simulink model "flc_case_3"  (R2018a)
settings: Solver=VariableStepAuto  StartTime=0.0  StopTime=30  RelTol=1e-3
libraries: fuzblock x1, simulink x1
settings Model: Creator=Lefteris  LastModifiedBy=Lefteris

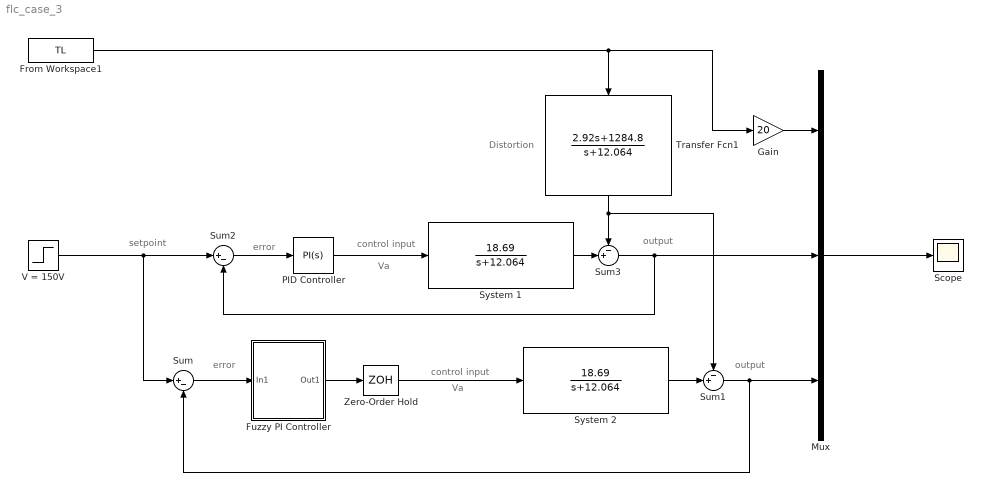
== system flc_case_3 ==
  note: Distortion
  note: setpoint
  note: output
  note: control input
  note: Va
  note: error
  note: error
  note: control input
  note: Va
  note: output
  From Workspace1 : FromWorkspace  VariableName=TL  SampleTime=0.01
  Fuzzy PI Controller : Subsystem
  Gain : Gain  Gain=20
  Mux : Mux  Inputs=3
  PID Controller : simulink/Continuous/PID Controller  Controller=PI  TimeDomain=Continuous-time  SampleTime=-1  IntegratorMethod=Forward Euler  FilterMethod=Forward Euler  Form=Parallel  UseFilter=on  ControllerParametersSource=internal  P=0.31011  I=8.1187  D=0  N=100  InitialConditionSource=internal  InitialConditionForIntegrator=0  InitialConditionForFilter=0  ExternalReset=none  LimitOutput=off  UpperSaturationLimit=inf  LowerSaturationLimit=-inf  LinearizeAsGain=on  AntiWindupMode=none  Kb=1  TrackingMode=off  Kt=1  PParamMin=[]  PParamMax=[]  IParamMin=[]  IParamMax=[]  DParamMin=[]  DParamMax=[]  NParamMin=[]  NParamMax=[]  KbParamMin=[]  KbParamMax=[]  KtParamMin=[]  KtParamMax=[]  POutMin=[]  POutMax=[]  IOutMin=[]  IOutMax=[]  DOutMin=[]  DOutMax=[]  NOutMin=[]  NOutMax=[]  KbOutMin=[]  KbOutMax=[]  KtOutMin=[]  KtOutMax=[]  IntegratorOutMin=[]  IntegratorOutMax=[]  FilterOutMin=[]  FilterOutMax=[]  SumOutMin=[]  SumOutMax=[]  SumI1OutMin=[]  SumI1OutMax=[]  SumI2OutMin=[]  SumI2OutMax=[]  SumI3OutMin=[]  SumI3OutMax=[]  SumDOutMin=[]  SumDOutMax=[]  SaturationOutMin=[]  SaturationOutMax=[]  IntegratorContinuousStateAttributes=''  IntegratorStateMustResolveToSignalObject=off  IntegratorRTWStateStorageClass=Auto  FilterContinuousStateAttributes=''  FilterStateMustResolveToSignalObject=off  FilterRTWStateStorageClass=Auto  DifferentiatorICPrevScaledInput=0  DifferentiatorOutMin=[]  DifferentiatorOutMax=[]  FilterDiffOutCoefMin=[]  FilterDiffOutCoefMax=[]  SumDenOutMin=[]  SumDenOutMax=[]  SumNumOutMin=[]  SumNumOutMax=[]  ReciprocalOutMin=[]  ReciprocalOutMax=[]  DivideOutMin=[]  DivideOutMax=[]  TunerSelectOption=Transfer Function Based (PID Tuner App)
  Scope : Scope
  Sum : Sum  Inputs=|+-
  Sum1 : Sum  Inputs=-+|
  Sum2 : Sum  Inputs=|+-
  Sum3 : Sum  Inputs=-+|
  System 1 : TransferFcn  Numerator=[18.69]  Denominator=[1 12.064]
  System 2 : TransferFcn  Numerator=[18.69]  Denominator=[1 12.064]
  Transfer Fcn1 : TransferFcn  Numerator=[2.92 1284.8]  Denominator=[1 12.064]
  V = 150V : Step  Time=0  After=150  SampleTime=0.01
  Zero-Order Hold : ZeroOrderHold  SampleTime=0.01
  wires:
  Zero-Order Hold/1 -> System 2/1
  Mux/1 -> Scope/1
  Sum/1 -> Fuzzy PI Controller/1(In1)
  V = 150V/1 -> Sum2/1, Sum/1
  Fuzzy PI Controller/1(Out1) -> Zero-Order Hold/1
  System 2/1 -> Sum1/2
  Sum1/1 -> Mux/3, Sum/2
  Sum2/1 -> PID Controller/1
  PID Controller/1 -> System 1/1
  System 1/1 -> Sum3/2
  Sum3/1 -> Sum2/2, Mux/2
  From Workspace1/1 -> Gain/1, Transfer Fcn1/1
  Gain/1 -> Mux/1
  Transfer Fcn1/1 -> Sum1/1, Sum3/1

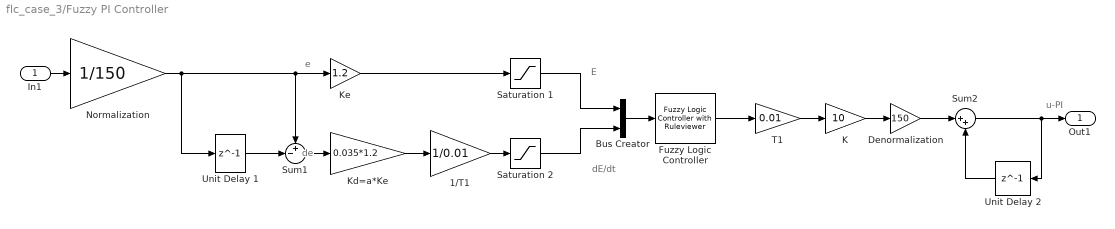
== system flc_case_3/Fuzzy PI Controller ==
  note: u-PI
  note: dE/dt
  note: E
  note: de
  note: e
  In1 : Inport
  1/T1 : Gain  Gain=1/0.01
  Bus Creator : BusCreator  Inputs=2
  "Denormalization " : Gain  Gain=150
  "Fuzzy Logic Controller " : fuzblock/Fuzzy Logic  Controller  with Ruleviewer  fismatrix=fis  Ts=1
  K : Gain  Gain=10
  Kd=a*Ke : Gain  Gain=0.035*1.2
  Ke : Gain  Gain=1.2
  Normalization : Gain  Gain=1/150
  "Saturation 1 " : Saturate  UpperLimit=1  LowerLimit=-1
  "Saturation 2 " : Saturate  UpperLimit=1  LowerLimit=-1
  Sum1 : Sum  Inputs=+-|
  Sum2 : Sum  Inputs=|++
  T1 : Gain  Gain=0.01
  Unit Delay 1 : Delay  DelayLength=1  SampleTime=0.01
  Unit Delay 2 : Delay  DelayLength=1  SampleTime=0.01
  Out1 : Outport
  wires:
  1/T1/1 -> "Saturation 2 "/1
  Kd=a*Ke/1 -> 1/T1/1
  Ke/1 -> "Saturation 1 "/1
  Sum1/1 -> Kd=a*Ke/1
  "Saturation 1 "/1 -> Bus Creator/1
  "Saturation 2 "/1 -> Bus Creator/2
  Unit Delay 2/1 -> Sum2/2
  K/1 -> "Denormalization "/1
  Normalization/1 -> Sum1/1, Ke/1, Unit Delay 1/1
  Unit Delay 1/1 -> Sum1/2
  T1/1 -> K/1
  "Denormalization "/1 -> Sum2/1
  Sum2/1 -> Unit Delay 2/1, Out1/1
  In1/1 -> Normalization/1
  "Fuzzy Logic Controller "/1 -> T1/1
  Bus Creator/1 -> "Fuzzy Logic Controller "/1
